simulink model "final_model_edited"  (R2015a)
settings: Solver=ode3  StartTime=0.0  StopTime=0  RelTol=1e-3
settings Model: Creator=BML  LastModifiedBy=BML
settings SolverCC: ZeroCrossAlgorithm=Adaptive  AutoInsertRateTranBlk=on
settings DebuggingCC: MaxConsecutiveZCsMsg=none

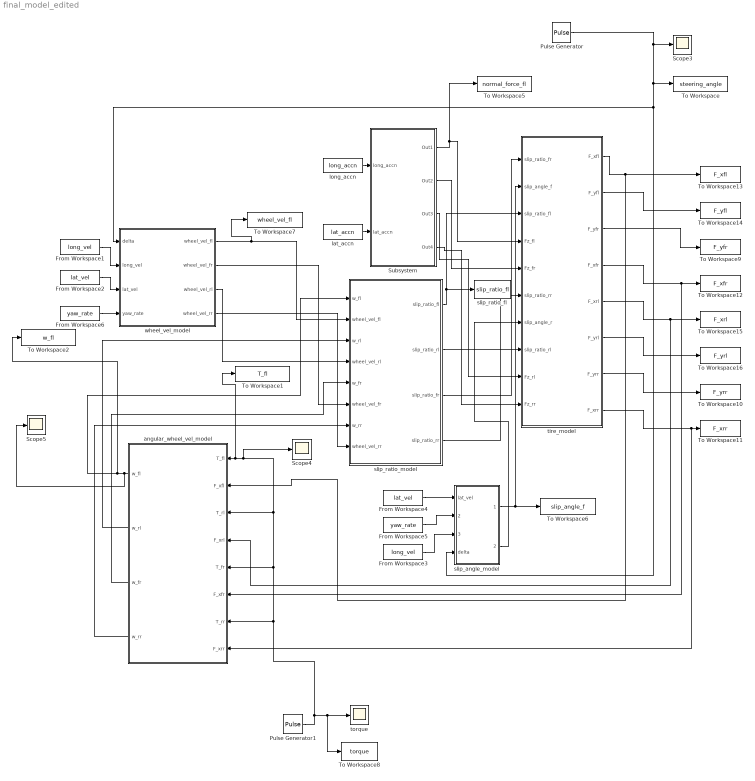
== system final_model_edited ==
  "           torque" : Scope
      settings: SaveName=ScopeData10
  From Workspace1 : FromWorkspace  VariableName=long_vel  SampleTime=1
  From Workspace2 : FromWorkspace  VariableName=lat_vel  SampleTime=1
  From Workspace3 : FromWorkspace  VariableName=long_vel  SampleTime=1
  From Workspace4 : FromWorkspace  VariableName=lat_vel  SampleTime=1
  From Workspace5 : FromWorkspace  VariableName=yaw_rate  SampleTime=1
  From Workspace6 : FromWorkspace  VariableName=yaw_rate  SampleTime=1
  Pulse Generator : DiscretePulseGenerator  PulseType=Time based  Amplitude=0  Period=8  PulseWidth=5  PhaseDelay=3
  Pulse Generator1 : DiscretePulseGenerator  PulseType=Time based  Amplitude=50  Period=8  PulseWidth=5  PhaseDelay=3
  Scope3 : Scope
      settings: SaveName=ScopeData3
  Scope4 : Scope
      settings: SaveName=ScopeData4
  Scope5 : Scope
      settings: SaveName=ScopeData5
  Subsystem : Subsystem
  To Workspace : ToWorkspace  VariableName=steering_angle  SaveFormat=Timeseries  SampleTime=1
  To Workspace1 : ToWorkspace  VariableName=T_fl  SaveFormat=Timeseries  SampleTime=1
  To Workspace10 : ToWorkspace  VariableName=F_yrr  SaveFormat=Timeseries  SampleTime=1
  To Workspace11 : ToWorkspace  VariableName=F_xrr  SaveFormat=Timeseries  SampleTime=1
  To Workspace12 : ToWorkspace  VariableName=F_xfr  SaveFormat=Timeseries  SampleTime=1
  To Workspace13 : ToWorkspace  VariableName=F_xfl  SaveFormat=Timeseries  SampleTime=1
  To Workspace14 : ToWorkspace  VariableName=F_yfl  SaveFormat=Timeseries  SampleTime=1
  To Workspace15 : ToWorkspace  VariableName=F_xrl  SaveFormat=Timeseries  SampleTime=1
  To Workspace16 : ToWorkspace  VariableName=F_yrl  SaveFormat=Timeseries  SampleTime=1
  To Workspace2 : ToWorkspace  VariableName=w_fl  SaveFormat=Timeseries  SampleTime=1
  To Workspace5 : ToWorkspace  VariableName=normal_force_fl  SaveFormat=Timeseries  SampleTime=1
  To Workspace6 : ToWorkspace  VariableName=slip_angle_f  SaveFormat=Timeseries  SampleTime=1
  To Workspace7 : ToWorkspace  VariableName=wheel_vel_fl  SaveFormat=Timeseries  SampleTime=1
  To Workspace8 : ToWorkspace  VariableName=torque  SaveFormat=Timeseries  SampleTime=-1
  To Workspace9 : ToWorkspace  VariableName=F_yfr  SaveFormat=Timeseries  SampleTime=1
  angular_wheel_vel_model : Subsystem
  lat_accn : FromWorkspace  VariableName=lat_accn  SampleTime=0
  long_accn : FromWorkspace  VariableName=long_accn  SampleTime=0
  slip_angle_model : Subsystem
  slip_ratio_fl : ToWorkspace  VariableName=slip_ratio_fl  SaveFormat=Timeseries  SampleTime=1
  slip_ratio_model : Subsystem
  tire_model : Subsystem
  wheel_vel_model : Subsystem
  wires:
  slip_ratio_model/1(slip_ratio_fl) -> slip_ratio_fl/1, tire_model/3(slip_ratio_fl)
  slip_ratio_model/2(slip_ratio_rl) -> tire_model/8(slip_ratio_rl)
  tire_model/2(F_yfl) -> To Workspace14/1
  Subsystem/1(Out1) -> To Workspace5/1, tire_model/4(Fz_fl)
  Subsystem/2(Out2) -> tire_model/5(Fz_fr)
  Subsystem/4(Out4) -> tire_model/10(Fz_rr)
  wheel_vel_model/3(wheel_vel_rl) -> slip_ratio_model/4(wheel_vel_rl)
  slip_ratio_model/3(slip_ratio_fr) -> tire_model/1(slip_ratio_fr)
  slip_ratio_model/4(slip_ratio_rr) -> tire_model/6(slip_ratio_rr)
  slip_angle_model/1(slip_angle_f) -> To Workspace6/1, tire_model/2("slip_angle_f  ")
  slip_angle_model/2(slip_angle_r) -> tire_model/7(slip_angle_r)
  wheel_vel_model/2(wheel_vel_fr) -> slip_ratio_model/6(wheel_vel_fr)
  wheel_vel_model/1(wheel_vel_fl) -> To Workspace7/1, slip_ratio_model/2(wheel_vel_fl)
  wheel_vel_model/4(wheel_vel_rr) -> slip_ratio_model/8(wheel_vel_rr)
  tire_model/1(F_xfl) -> angular_wheel_vel_model/2(F_xfl), To Workspace13/1
  angular_wheel_vel_model/1(w_fl) -> slip_ratio_model/1(w_fl), To Workspace2/1, Scope5/1
  angular_wheel_vel_model/2(w_rl) -> slip_ratio_model/3(w_rl)
  angular_wheel_vel_model/3(w_fr) -> slip_ratio_model/5(w_fr)
  angular_wheel_vel_model/4(w_rr) -> slip_ratio_model/7(w_rr)
  Pulse Generator/1 -> To Workspace/1, slip_angle_model/4(delta), wheel_vel_model/1(delta), Scope3/1
  Pulse Generator1/1 -> To Workspace8/1, "           torque"/1, angular_wheel_vel_model/7(T_rr), angular_wheel_vel_model/5(T_fr), angular_wheel_vel_model/3(T_rl), Scope4/1, To Workspace1/1, angular_wheel_vel_model/1(T_fl)
  Subsystem/3(Out3) -> tire_model/9(Fz_rl)
  tire_model/3(F_yfr) -> To Workspace9/1
  tire_model/4(F_xfr) -> angular_wheel_vel_model/6(F_xfr), To Workspace12/1
  tire_model/6(F_yrl) -> To Workspace16/1
  tire_model/7(F_yrr) -> To Workspace10/1
  tire_model/8(F_xrr) -> angular_wheel_vel_model/8(F_xrr), To Workspace11/1
  long_accn/1 -> Subsystem/1(long_accn)
  lat_accn/1 -> Subsystem/2(lat_accn)
  From Workspace5/1 -> slip_angle_model/2(yaw_rate)
  tire_model/5(F_xrl) -> To Workspace15/1, angular_wheel_vel_model/4(F_xrl)
  From Workspace4/1 -> slip_angle_model/1(lat_vel)
  From Workspace3/1 -> slip_angle_model/3(long_vel)
  From Workspace1/1 -> wheel_vel_model/2(long_vel)
  From Workspace2/1 -> wheel_vel_model/3(lat_vel)
  From Workspace6/1 -> wheel_vel_model/4(yaw_rate)

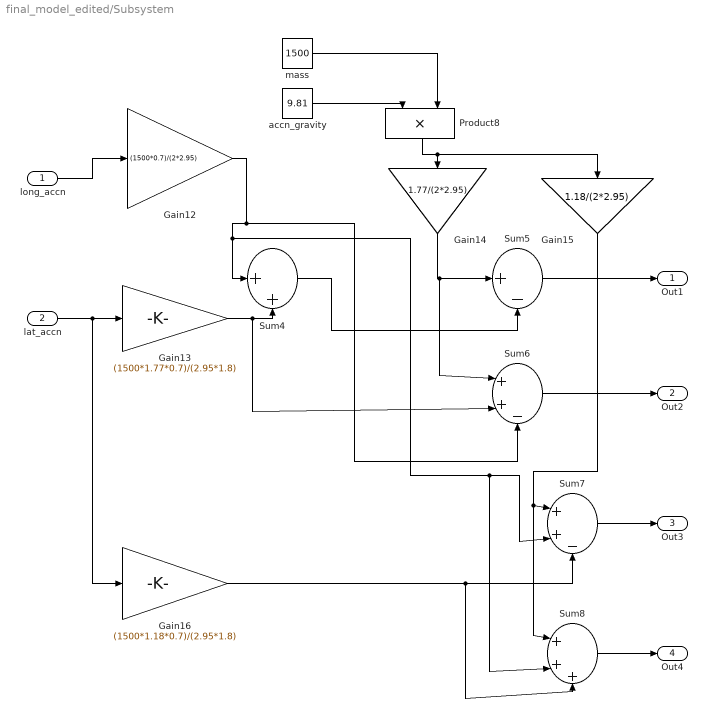
== system final_model_edited/Subsystem ==
  long_accn : Inport
  lat_accn : Inport  Port=2
  Gain12 : Gain  Gain=(1500*0.7)/(2*2.95)
  Gain13 : Gain  Gain=(1500*1.77*0.7)/(2.95*1.8)
  Gain14 : Gain  Gain=1.77/(2*2.95)
  Gain15 : Gain  Gain=1.18/(2*2.95)
  Gain16 : Gain  Gain=(1500*1.18*0.7)/(2.95*1.8)
  Product8 : Product
  Sum4 : Sum  Inputs=|++
  Sum5 : Sum  Inputs=|+-
  Sum6 : Sum  Inputs=|++-
  Sum7 : Sum  Inputs=|++-
  Sum8 : Sum  Inputs=|+++
  "accn_gravity " : Constant  Value=9.81
  mass : Constant  Value=1500
  Out1 : Outport
  Out2 : Outport  Port=2
  Out3 : Outport  Port=3
  Out4 : Outport  Port=4
  wires:
  Gain12/1 -> Sum4/1, Sum8/2, Sum7/2, Sum6/3
  Gain15/1 -> Sum8/1, Sum7/1
  Gain16/1 -> Sum8/3, Sum7/3
  Sum7/1 -> Out3/1
  lat_accn/1 -> Gain16/1, Gain13/1
  Gain13/1 -> Sum6/2, Sum4/2
  Sum5/1 -> Out1/1
  Sum6/1 -> Out2/1
  Sum4/1 -> Sum5/2
  long_accn/1 -> Gain12/1
  mass/1 -> Product8/2
  Gain14/1 -> Sum5/1, Sum6/1
  Sum8/1 -> Out4/1
  Product8/1 -> Gain15/1, Gain14/1
  "accn_gravity "/1 -> Product8/1

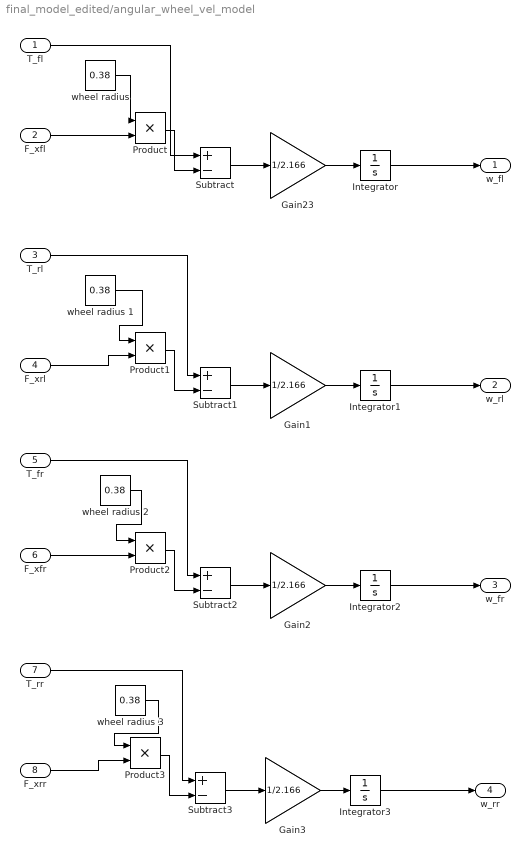
== system final_model_edited/angular_wheel_vel_model ==
  T_fl : Inport
  F_xfl : Inport  Port=2
  T_rl : Inport  Port=3
  F_xrl : Inport  Port=4
  T_fr : Inport  Port=5
  F_xfr : Inport  Port=6
  T_rr : Inport  Port=7
  F_xrr : Inport  Port=8
  Gain{1..3,23} (4 alike) : Gain  Gain=1/2.166
  Integrator{,1..3} (4 alike) : Integrator  InitialCondition=58.5
  Product{,1..3} (4 alike) : Product
  Subtract{,1..3} (4 alike) : Sum  Inputs=+-
  wheel radius {,1..3} (4 alike) : Constant  Value=0.38
  w_fl : Outport
  w_rl : Outport  Port=2
  w_fr : Outport  Port=3
  w_rr : Outport  Port=4
  wires:
  Gain23/1 -> Integrator/1
  Integrator/1 -> w_fl/1
  F_xfl/1 -> Product/2
  Product/1 -> Subtract/2
  wheel radius 1/1 -> Product1/1
  T_rl/1 -> Subtract1/1
  T_fl/1 -> Subtract/1
  Subtract/1 -> Gain23/1
  F_xrl/1 -> Product1/2
  "wheel radius "/1 -> Product/1
  Subtract2/1 -> Gain2/1
  wheel radius 2/1 -> Product2/1
  Product1/1 -> Subtract1/2
  F_xrr/1 -> Product3/2
  T_rr/1 -> Subtract3/1
  Gain3/1 -> Integrator3/1
  Subtract1/1 -> Gain1/1
  Gain1/1 -> Integrator1/1
  Gain2/1 -> Integrator2/1
  Subtract3/1 -> Gain3/1
  Integrator3/1 -> w_rr/1
  wheel radius 3/1 -> Product3/1
  F_xfr/1 -> Product2/2
  Product3/1 -> Subtract3/2
  T_fr/1 -> Subtract2/1
  Product2/1 -> Subtract2/2
  Integrator1/1 -> w_rl/1
  Integrator2/1 -> w_fr/1

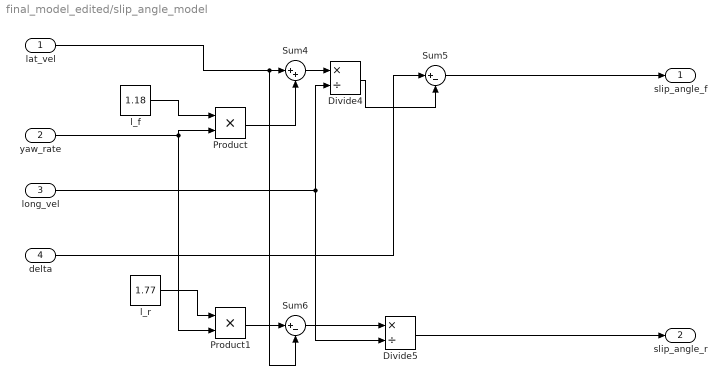
== system final_model_edited/slip_angle_model ==
  lat_vel : Inport
  yaw_rate : Inport  Port=2
  long_vel : Inport  Port=3
  delta : Inport  Port=4
  Divide4 : Product  Inputs=*/
  Divide5 : Product  Inputs=*/
  Product : Product
  Product1 : Product
  Sum4 : Sum  Inputs=|++
  Sum5 : Sum  Inputs=|+-
  Sum6 : Sum  Inputs=|+-
  l_f : Constant  Value=1.18
  l_r : Constant  Value=1.77
  slip_angle_f : Outport
  slip_angle_r : Outport  Port=2
  wires:
  yaw_rate/1 -> Product1/2, Product/2
  long_vel/1 -> Divide5/2, Divide4/2
  l_f/1 -> Product/1
  lat_vel/1 -> Sum6/2, Sum4/1
  Divide4/1 -> Sum5/2
  Product/1 -> Sum4/2
  Sum4/1 -> Divide4/1
  Divide5/1 -> slip_angle_r/1
  delta/1 -> Sum5/1
  Sum5/1 -> slip_angle_f/1
  Product1/1 -> Sum6/1
  l_r/1 -> Product1/1
  Sum6/1 -> Divide5/1

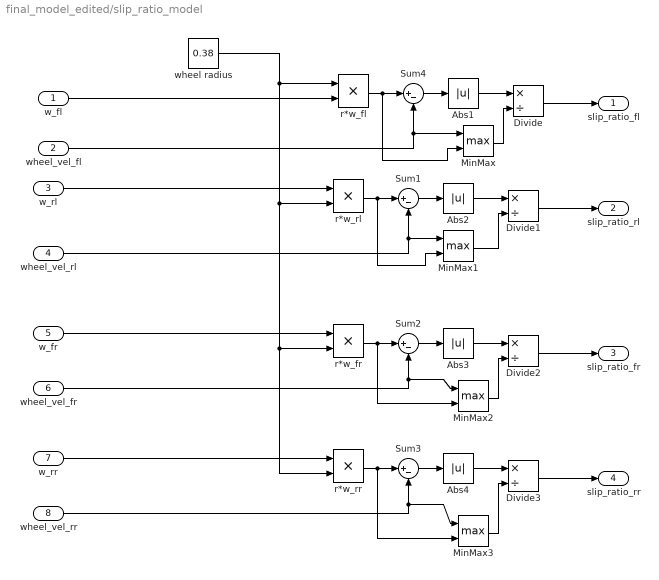
== system final_model_edited/slip_ratio_model ==
  w_fl : Inport
  wheel_vel_fl : Inport  Port=2
  w_rl : Inport  Port=3
  wheel_vel_rl : Inport  Port=4
  w_fr : Inport  Port=5
  wheel_vel_fr : Inport  Port=6
  w_rr : Inport  Port=7
  wheel_vel_rr : Inport  Port=8
  Abs{1..4} (4 alike) : Abs
  Divide{,1..3} (4 alike) : Product  Inputs=*/
  MinMax{,1..3} (4 alike) : MinMax  Function=max  Inputs=2
  Sum{1..4} (4 alike) : Sum  Inputs=|+-
  r*w_fl : Product  Inputs=**
  r*w_fr : Product  Inputs=**
  r*w_rl : Product  Inputs=**
  r*w_rr : Product  Inputs=**
  wheel radius : Constant  Value=0.38
  slip_ratio_fl : Outport
  slip_ratio_rl : Outport  Port=2
  slip_ratio_fr : Outport  Port=3
  slip_ratio_rr : Outport  Port=4
  wires:
  w_fl/1 -> r*w_fl/2
  r*w_fl/1 -> MinMax/2, Sum4/1
  wheel radius/1 -> r*w_fl/1, r*w_rl/2, r*w_rr/2, r*w_fr/2
  wheel_vel_fl/1 -> Sum4/2, MinMax/1
  Sum4/1 -> Abs1/1
  Abs1/1 -> Divide/1
  MinMax/1 -> Divide/2
  Divide/1 -> slip_ratio_fl/1
  r*w_rl/1 -> MinMax1/2, Sum1/1
  wheel_vel_rl/1 -> Sum1/2, MinMax1/1
  Sum1/1 -> Abs2/1
  Abs2/1 -> Divide1/1
  MinMax1/1 -> Divide1/2
  Divide1/1 -> slip_ratio_rl/1
  w_rl/1 -> r*w_rl/1
  r*w_fr/1 -> MinMax2/2, Sum2/1
  wheel_vel_fr/1 -> MinMax2/1, Sum2/2
  Sum2/1 -> Abs3/1
  Abs3/1 -> Divide2/1
  MinMax2/1 -> Divide2/2
  Divide2/1 -> slip_ratio_fr/1
  w_fr/1 -> r*w_fr/1
  r*w_rr/1 -> MinMax3/2, Sum3/1
  wheel_vel_rr/1 -> MinMax3/1, Sum3/2
  Sum3/1 -> Abs4/1
  Abs4/1 -> Divide3/1
  MinMax3/1 -> Divide3/2
  Divide3/1 -> slip_ratio_rr/1
  w_rr/1 -> r*w_rr/1

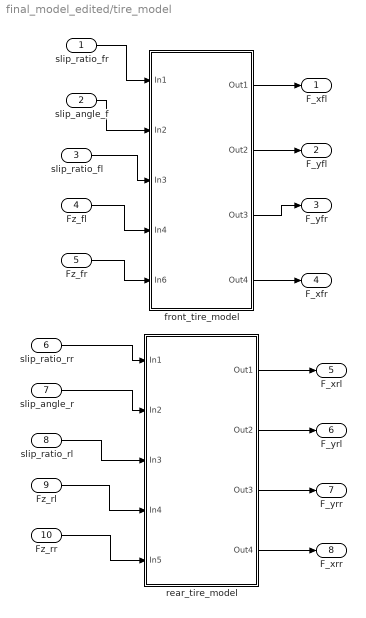
== system final_model_edited/tire_model ==
  slip_ratio_fr : Inport
  "slip_angle_f  " : Inport  Port=2
  slip_ratio_fl : Inport  Port=3
  Fz_fl : Inport  Port=4
  Fz_fr : Inport  Port=5
  slip_ratio_rr : Inport  Port=6
  slip_angle_r : Inport  Port=7
  slip_ratio_rl : Inport  Port=8
  Fz_rl : Inport  Port=9
  Fz_rr : Inport  Port=10
  front_tire_model : Subsystem
  rear_tire_model : Subsystem
  F_xfl : Outport
  F_yfl : Outport  Port=2
  F_yfr : Outport  Port=3
  F_xfr : Outport  Port=4
  F_xrl : Outport  Port=5
  F_yrl : Outport  Port=6
  F_yrr : Outport  Port=7
  F_xrr : Outport  Port=8
  wires:
  slip_ratio_rr/1 -> rear_tire_model/1(In1)
  slip_angle_r/1 -> rear_tire_model/2(In2)
  rear_tire_model/3(Out3) -> F_yrr/1
  slip_ratio_rl/1 -> rear_tire_model/3(In3)
  rear_tire_model/2(Out2) -> F_yrl/1
  Fz_rr/1 -> rear_tire_model/5(In5)
  rear_tire_model/1(Out1) -> F_xrl/1
  rear_tire_model/4(Out4) -> F_xrr/1
  Fz_rl/1 -> rear_tire_model/4(In4)
  "slip_angle_f  "/1 -> front_tire_model/2(In2)
  slip_ratio_fr/1 -> front_tire_model/1(In1)
  slip_ratio_fl/1 -> front_tire_model/3(In3)
  Fz_fr/1 -> front_tire_model/5(In6)
  front_tire_model/1(Out1) -> F_xfl/1
  front_tire_model/3(Out3) -> F_yfr/1
  front_tire_model/2(Out2) -> F_yfl/1
  Fz_fl/1 -> front_tire_model/4(In4)
  front_tire_model/4(Out4) -> F_xfr/1

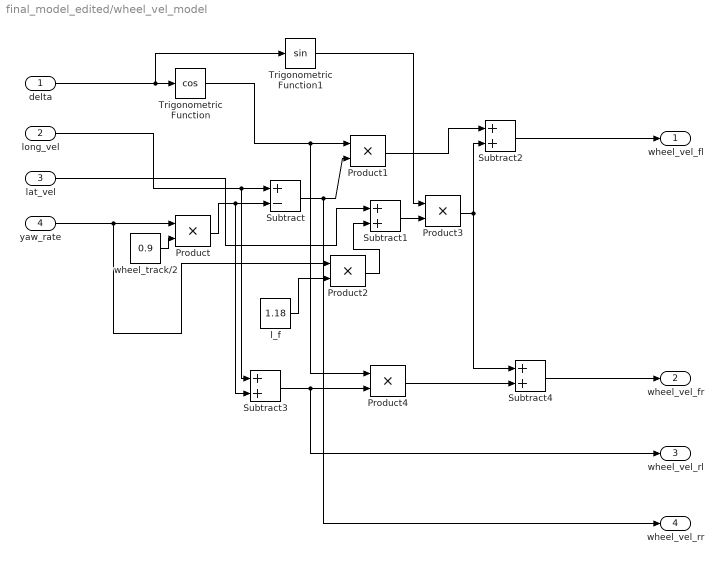
== system final_model_edited/wheel_vel_model ==
  delta : Inport
  long_vel : Inport  Port=2
  lat_vel : Inport  Port=3
  yaw_rate : Inport  Port=4
  Product{,1..4} (5 alike) : Product
  Subtract : Sum  Inputs=+-
  Subtract{1..4} (4 alike) : Sum
  Trigonometric Function : Trigonometry  Operator=cos
  Trigonometric Function1 : Trigonometry
  l_f : Constant  Value=1.18
  wheel_track/2 : Constant  Value=0.9
  wheel_vel_fl : Outport
  wheel_vel_fr : Outport  Port=2
  wheel_vel_rl : Outport  Port=3
  wheel_vel_rr : Outport  Port=4
  wires:
  long_vel/1 -> Subtract3/1, Subtract/1
  l_f/1 -> Product2/2
  Subtract3/1 -> wheel_vel_rl/1, Product4/2
  Trigonometric Function/1 -> Product4/1, Product1/1
  Subtract1/1 -> Product3/2
  Subtract/1 -> wheel_vel_rr/1, Product1/2
  Product4/1 -> Subtract4/2
  Subtract4/1 -> wheel_vel_fr/1
  lat_vel/1 -> Subtract1/1
  Product/1 -> Subtract3/2, Subtract/2
  Product2/1 -> Subtract1/2
  Product1/1 -> Subtract2/1
  yaw_rate/1 -> Product/1, Product2/1
  wheel_track/2/1 -> Product/2
  Trigonometric Function1/1 -> Product3/1
  Subtract2/1 -> wheel_vel_fl/1
  delta/1 -> Trigonometric Function1/1, Trigonometric Function/1
  Product3/1 -> Subtract2/2, Subtract4/1

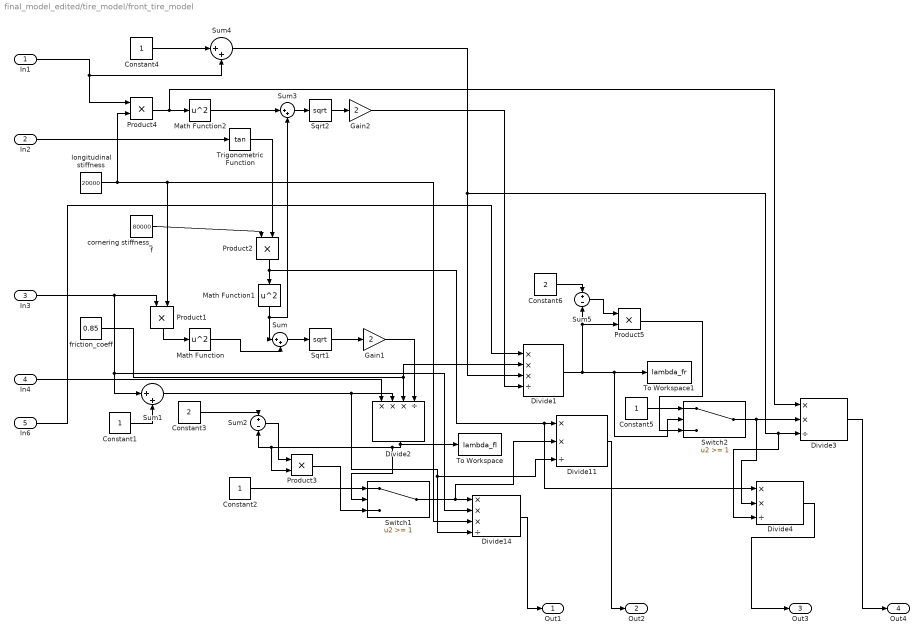
== system final_model_edited/tire_model/front_tire_model ==
  In1 : Inport
  In2 : Inport  Port=2
  In3 : Inport  Port=3
  In4 : Inport  Port=4
  In6 : Inport  Port=5
  Constant{1..2,4..5} (4 alike) : Constant
  Constant3 : Constant  Value=2
  Constant6 : Constant  Value=2
  Divide1 : Product  Inputs=***/
  Divide11 : Product  Inputs=**/
  Divide14 : Product  Inputs=***/
  Divide2 : Product  Inputs=***/
  Divide3 : Product  Inputs=**/
  Divide4 : Product  Inputs=**/
  Gain1 : Gain  Gain=2
  Gain2 : Gain  Gain=2
  Math Function : Math  Operator=square  SaturateOnIntegerOverflow=on
  Math Function1 : Math  Operator=square  SaturateOnIntegerOverflow=on
  Math Function2 : Math  Operator=square  SaturateOnIntegerOverflow=on
  Product{1..5} (5 alike) : Product
  Sqrt1 : Sqrt  SaturateOnIntegerOverflow=on
  Sqrt2 : Sqrt  SaturateOnIntegerOverflow=on
  Sum{,1,3..4} (4 alike) : Sum  Inputs=|++
  Sum2 : Sum  Inputs=+-
  Sum5 : Sum  Inputs=+-
  Switch1 : Switch  Threshold=1
  Switch2 : Switch  Threshold=1
  To Workspace : ToWorkspace  VariableName=lambda_fl  SaveFormat=Timeseries  SampleTime=-1
  To Workspace1 : ToWorkspace  VariableName=lambda_fr  SaveFormat=Timeseries  SampleTime=-1
  Trigonometric Function : Trigonometry  Operator=tan
  cornering stiffness_f : Constant  Value=80000
  friction_coeff : Constant  Value=0.85
  longitudinal stiffness : Constant  Value=20000
  Out1 : Outport
  Out2 : Outport  Port=2
  Out3 : Outport  Port=3
  Out4 : Outport  Port=4
  wires:
  Math Function/1 -> Sum/2
  Constant1/1 -> Sum1/2
  Gain1/1 -> Divide2/4
  Trigonometric Function/1 -> Product2/2
  In3/1 -> Divide14/2, Sum1/1, Product1/1
  Sum/1 -> Sqrt1/1
  friction_coeff/1 -> Divide1/2, Divide2/3
  Sqrt1/1 -> Gain1/1
  In4/1 -> Divide2/1
  Product3/1 -> Switch1/3
  Gain2/1 -> Divide1/4
  Math Function1/1 -> Sum3/2, Sum/1
  Sum5/1 -> Product5/1
  Product2/1 -> Divide4/1, Divide11/1, Math Function1/1
  Constant5/1 -> Switch2/1
  cornering stiffness_f/1 -> Product2/1
  Switch2/1 -> Divide4/2, Divide3/2
  Divide14/1 -> Out1/1
  In6/1 -> Divide1/1
  Sum4/1 -> Divide4/3, Divide3/3, Divide1/3
  Constant2/1 -> Switch1/1
  Sum1/1 -> Divide11/3, Divide14/4, Divide2/2
  Divide11/1 -> Out2/1
  In1/1 -> Sum4/2, Product4/1
  Switch1/1 -> Divide11/2, Divide14/1
  Constant4/1 -> Sum4/1
  longitudinal stiffness/1 -> Product4/2, Product1/2, Divide14/3
  Sum3/1 -> Sqrt2/1
  Math Function2/1 -> Sum3/1
  Constant6/1 -> Sum5/1
  Sqrt2/1 -> Gain2/1
  Product4/1 -> Divide3/1, Math Function2/1
  Divide3/1 -> Out4/1
  Divide4/1 -> Out3/1
  Sum2/1 -> Product3/1
  Divide1/1 -> Switch2/2, To Workspace1/1, Sum5/2, Product5/2
  Constant3/1 -> Sum2/1
  Product1/1 -> Math Function/1
  In2/1 -> Trigonometric Function/1
  Divide2/1 -> Switch1/2, Product3/2, Sum2/2, To Workspace/1
  Product5/1 -> Switch2/3

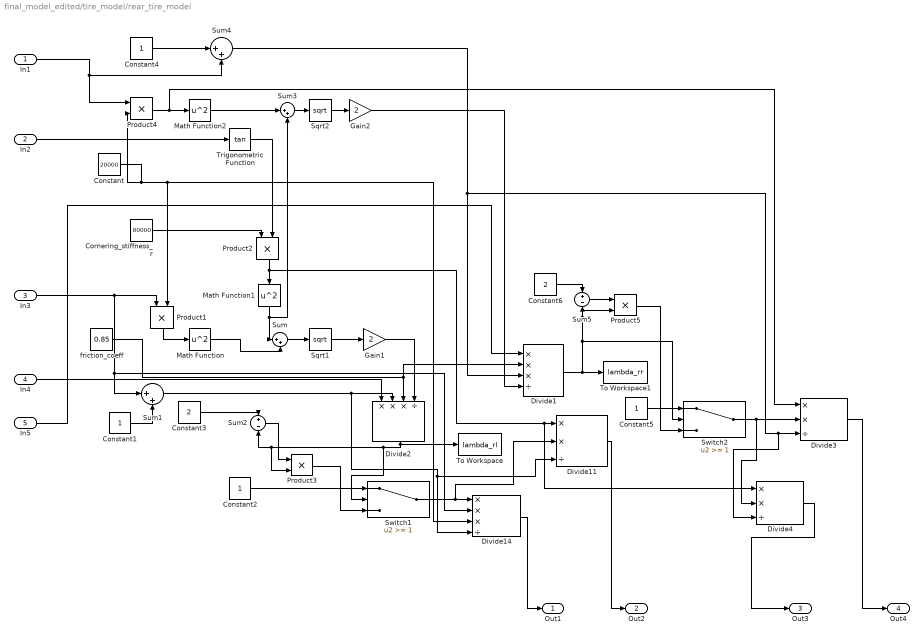
== system final_model_edited/tire_model/rear_tire_model ==
  In1 : Inport
  In2 : Inport  Port=2
  In3 : Inport  Port=3
  In4 : Inport  Port=4
  In5 : Inport  Port=5
  Constant : Constant  Value=20000
  Constant{1..2,4..5} (4 alike) : Constant
  Constant3 : Constant  Value=2
  Constant6 : Constant  Value=2
  Cornering_stiffness_r : Constant  Value=80000
  Divide1 : Product  Inputs=***/
  Divide11 : Product  Inputs=**/
  Divide14 : Product  Inputs=***/
  Divide2 : Product  Inputs=***/
  Divide3 : Product  Inputs=**/
  Divide4 : Product  Inputs=**/
  Gain1 : Gain  Gain=2
  Gain2 : Gain  Gain=2
  Math Function : Math  Operator=square  SaturateOnIntegerOverflow=on
  Math Function1 : Math  Operator=square  SaturateOnIntegerOverflow=on
  Math Function2 : Math  Operator=square  SaturateOnIntegerOverflow=on
  Product{1..5} (5 alike) : Product
  Sqrt1 : Sqrt  SaturateOnIntegerOverflow=on
  Sqrt2 : Sqrt  SaturateOnIntegerOverflow=on
  Sum{,1,3..4} (4 alike) : Sum  Inputs=|++
  Sum2 : Sum  Inputs=+-
  Sum5 : Sum  Inputs=+-
  Switch1 : Switch  Threshold=1
  Switch2 : Switch  Threshold=1
  To Workspace : ToWorkspace  VariableName=lambda_rl  SaveFormat=Timeseries  SampleTime=-1
  To Workspace1 : ToWorkspace  VariableName=lambda_rr  SaveFormat=Timeseries  SampleTime=-1
  Trigonometric Function : Trigonometry  Operator=tan
  friction_coeff : Constant  Value=0.85
  Out1 : Outport
  Out2 : Outport  Port=2
  Out3 : Outport  Port=3
  Out4 : Outport  Port=4
  wires:
  Sum2/1 -> Product3/1
  In4/1 -> Divide2/1
  Divide2/1 -> Switch1/2, Product3/2, Sum2/2, To Workspace/1
  Product3/1 -> Switch1/3
  Constant3/1 -> Sum2/1
  Constant2/1 -> Switch1/1
  friction_coeff/1 -> Divide1/2, Divide2/3
  Sum1/1 -> Divide11/3, Divide14/4, Divide2/2
  Constant/1 -> Product4/2, Product1/2, Divide14/3
  Divide14/1 -> Out1/1
  Gain1/1 -> Divide2/4
  Constant4/1 -> Sum4/1
  Product2/1 -> Divide4/1, Divide11/1, Math Function1/1
  Sum3/1 -> Sqrt2/1
  Sqrt2/1 -> Gain2/1
  Gain2/1 -> Divide1/4
  In1/1 -> Sum4/2, Product4/1
  Math Function2/1 -> Sum3/1
  Sum5/1 -> Product5/1
  Divide11/1 -> Out2/1
  In5/1 -> Divide1/1
  Math Function1/1 -> Sum3/2, Sum/1
  Cornering_stiffness_r/1 -> Product2/1
  Switch1/1 -> Divide11/2, Divide14/1
  Divide1/1 -> Switch2/2, Product5/2, Sum5/2, To Workspace1/1
  Constant6/1 -> Sum5/1
  In3/1 -> Divide14/2, Sum1/1, Product1/1
  Product1/1 -> Math Function/1
  Trigonometric Function/1 -> Product2/2
  Sum/1 -> Sqrt1/1
  Sqrt1/1 -> Gain1/1
  Constant1/1 -> Sum1/2
  In2/1 -> Trigonometric Function/1
  Math Function/1 -> Sum/2
  Constant5/1 -> Switch2/1
  Product4/1 -> Divide3/1, Math Function2/1
  Product5/1 -> Switch2/3
  Switch2/1 -> Divide4/2, Divide3/2
  Divide4/1 -> Out3/1
  Sum4/1 -> Divide4/3, Divide3/3, Divide1/3
  Divide3/1 -> Out4/1
